simulink model "PrevVersion"  (R2020a)
settings: Solver=VariableStepAuto  StartTime=0.0  StopTime=10.0  RelTol=1e-3
libraries: simulink x3
settings Model: Creator=99003752  LastModifiedBy=99003752

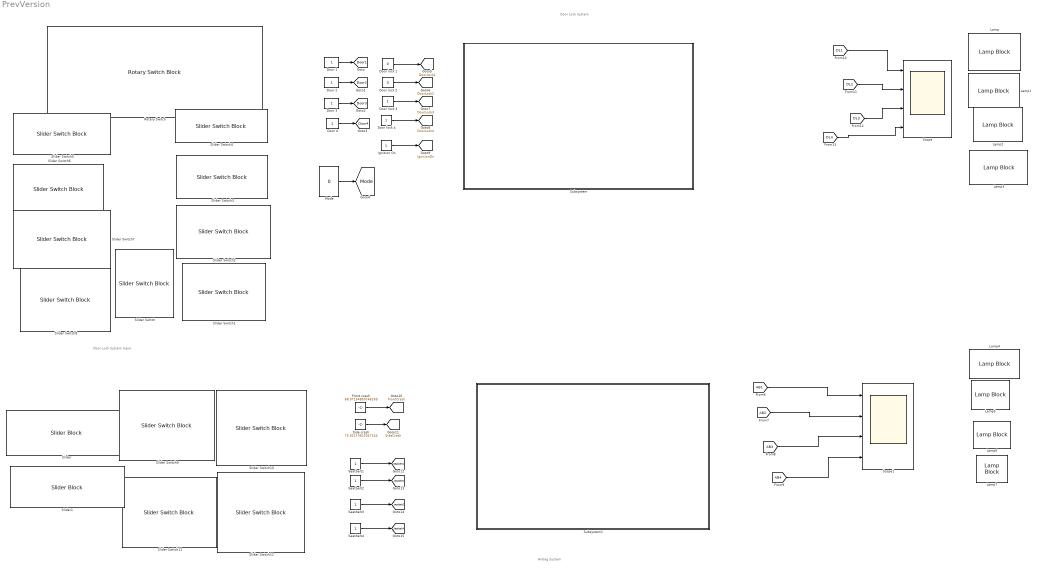
== system PrevVersion ==
  note: Door Lock System
  note: Airbag System
  note: Door Lock System Input
  Door {1..4} (4 alike) : Constant
  Door lock 1 : Constant  Value=0
  Door lock 2 : Constant  Value=0
  Door lock 3 : Constant
  Door lock 4 : Constant
  Front crash : Constant  Value=68.97154850746269
  Ignition On : Constant
  Lamp{,1..7} (8 alike) : LampBlock
  Mode : Constant  Value=0
  Rotary Switch : RotarySwitchBlock
      settings: Values={{'Off', 'Automatic Lock', 'Lock Out Protection', 'Driver Control'}, [0 1 2 3]}
  Scope : Scope  NumInputPorts=4
  Scope1 : Scope  NumInputPorts=4
  Seatbelt{1..4} (4 alike) : Constant
  Side crash : Constant  Value=75.92273622047244
  Slider : SliderBlock
  Slider Switch{,1..12} (13 alike) : SliderSwitchBlock
      settings: Values={{'Off', 'On'}, [0 1]}
  Slider1 : SliderBlock
  Subsystem : Subsystem
  Subsystem1 : Subsystem
  tag scope: Door1=global, Door2=global, Door3=global, Door4=global, DoorLock1=global, DoorLock2=global, DoorLock3=global, DoorLock4=global, FrontCrash=global, IgnitionOn=global, Mode=global, Seatbelt1=global, Seatbelt4=global, SideCrash=global, seatbelt2=global, seatbelt3=global
  wires:
  [DL4] -> Scope/4
  [DL1] -> Scope/1
  Door lock 1/1 -> [DoorLock1]
  Seatbelt1/1 -> [Seatbelt1]
  Ignition On/1 -> [IgnitionOn]
  Door lock 2/1 -> [DoorLock2]
  Door 2/1 -> [Door2]
  Door 3/1 -> [Door3]
  Seatbelt4/1 -> [Seatbelt4]
  Door lock 4/1 -> [DoorLock4]
  [DL2] -> Scope/2
  Mode/1 -> [Mode]
  Seatbelt2/1 -> [seatbelt2]
  Door 4/1 -> [Door4]
  Door lock 3/1 -> [DoorLock3]
  Seatbelt3/1 -> [seatbelt3]
  Side crash/1 -> [SideCrash]
  Front crash/1 -> [FrontCrash]
  [AB1] -> Scope1/1
  [AB2] -> Scope1/2
  Door 1/1 -> [Door1]
  [AB3] -> Scope1/3
  [DL3] -> Scope/3
  [AB4] -> Scope1/4

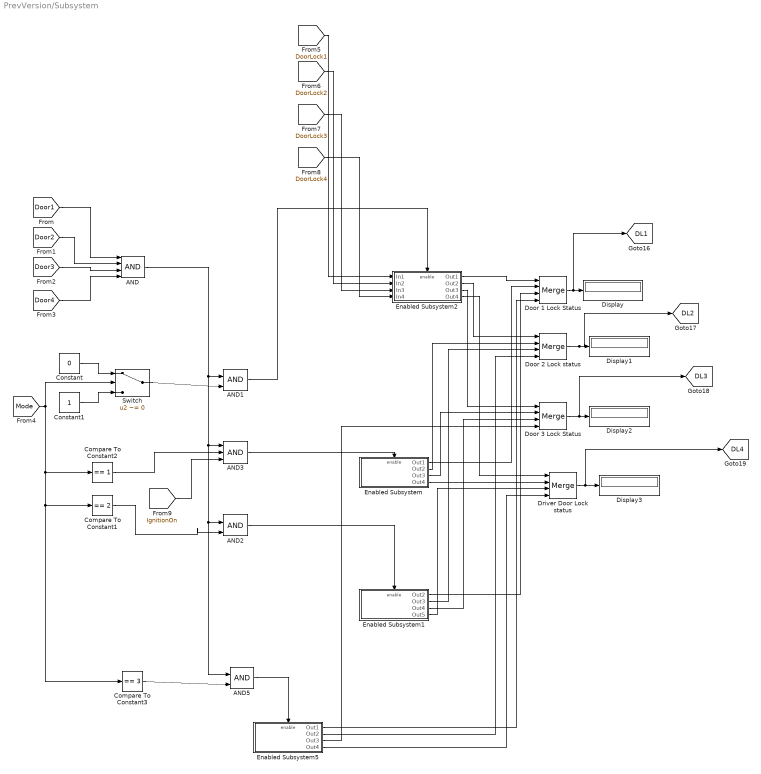
== system PrevVersion/Subsystem ==
  AND : Logic  Inputs=4  IconShape=distinctive  AllPortsSameDT=off  OutDataTypeStr=boolean
  AND1 : Logic  IconShape=distinctive  AllPortsSameDT=off  OutDataTypeStr=boolean
  AND2 : Logic  IconShape=distinctive  AllPortsSameDT=off  OutDataTypeStr=boolean
  AND3 : Logic  Inputs=3  IconShape=distinctive  AllPortsSameDT=off  OutDataTypeStr=boolean
  AND5 : Logic  IconShape=distinctive  AllPortsSameDT=off  OutDataTypeStr=boolean
  Compare To Constant1 : simulink/Logic and Bit Operations/Compare To Constant  relop===  const=2  OutDataTypeStr=boolean
  Compare To Constant2 : simulink/Logic and Bit Operations/Compare To Constant  relop===  const=1  OutDataTypeStr=boolean
  Compare To Constant3 : simulink/Logic and Bit Operations/Compare To Constant  relop===  const=3  OutDataTypeStr=boolean
  Constant : Constant  Value=0
  Constant1 : Constant
  Display{,1..3} (4 alike) : Display
  Door 1 Lock Status : Merge  Inputs=4
  Door 2 Lock status : Merge  Inputs=4
  Door 3 Lock Status : Merge  Inputs=4
  "Driver Door Lock status " : Merge  Inputs=4
  Enabled Subsystem : Subsystem  TreatAsAtomicUnit=on
  Enabled Subsystem1 : Subsystem  TreatAsAtomicUnit=on
  Enabled Subsystem2 : Subsystem  TreatAsAtomicUnit=on
  Enabled Subsystem5 : Subsystem  TreatAsAtomicUnit=on
  Switch : Switch  Criteria=u2 ~= 0
  tag scope: DL1=global, DL2=global, DL3=global, DL4=global
  wires:
  Door 1 Lock Status/1 -> [DL1], Display/1
  AND/1 -> AND5/1, AND2/1, AND3/1, AND1/1
  "Driver Door Lock status "/1 -> [DL4], Display3/1
  Door 2 Lock status/1 -> [DL2], Display1/1
  [Door4] -> AND/4
  [Mode] -> Switch/2, Compare To Constant2/1, Compare To Constant1/1, Compare To Constant3/1
  Door 3 Lock Status/1 -> [DL3], Display2/1
  Enabled Subsystem5/1(Out1) -> Door 1 Lock Status/4
  Enabled Subsystem5/2(Out2) -> Door 2 Lock status/4
  AND5/1 -> Enabled Subsystem5/Enable
  [DoorLock3] -> Enabled Subsystem2/3(In3)
  [IgnitionOn] -> AND3/3
  Enabled Subsystem1/4(Out5) -> "Driver Door Lock status "/3
  [Door1] -> AND/1
  [DoorLock4] -> Enabled Subsystem2/4(In4)
  [Door3] -> AND/3
  Enabled Subsystem2/4(Out4) -> "Driver Door Lock status "/1
  [DoorLock1] -> Enabled Subsystem2/1(In1)
  AND2/1 -> Enabled Subsystem1/Enable
  Enabled Subsystem5/3(Out3) -> Door 3 Lock Status/4
  Enabled Subsystem2/3(Out3) -> Door 3 Lock Status/1
  Enabled Subsystem5/4(Out4) -> "Driver Door Lock status "/4
  Enabled Subsystem/1(Out1) -> Door 1 Lock Status/2
  Compare To Constant3/1 -> AND5/2
  Enabled Subsystem1/2(Out3) -> Door 2 Lock status/3
  Enabled Subsystem1/1(Out2) -> Door 1 Lock Status/3
  Constant/1 -> Switch/1
  Enabled Subsystem/2(Out2) -> Door 2 Lock status/2
  Constant1/1 -> Switch/3
  AND3/1 -> Enabled Subsystem/Enable
  [Door2] -> AND/2
  Enabled Subsystem2/2(Out2) -> Door 2 Lock status/1
  Switch/1 -> AND1/2
  Enabled Subsystem/4(Out4) -> "Driver Door Lock status "/2
  Enabled Subsystem2/1(Out1) -> Door 1 Lock Status/1
  Enabled Subsystem/3(Out3) -> Door 3 Lock Status/2
  Enabled Subsystem1/3(Out4) -> Door 3 Lock Status/3
  [DoorLock2] -> Enabled Subsystem2/2(In2)
  AND1/1 -> Enabled Subsystem2/Enable
  Compare To Constant1/1 -> AND2/2
  Compare To Constant2/1 -> AND3/2

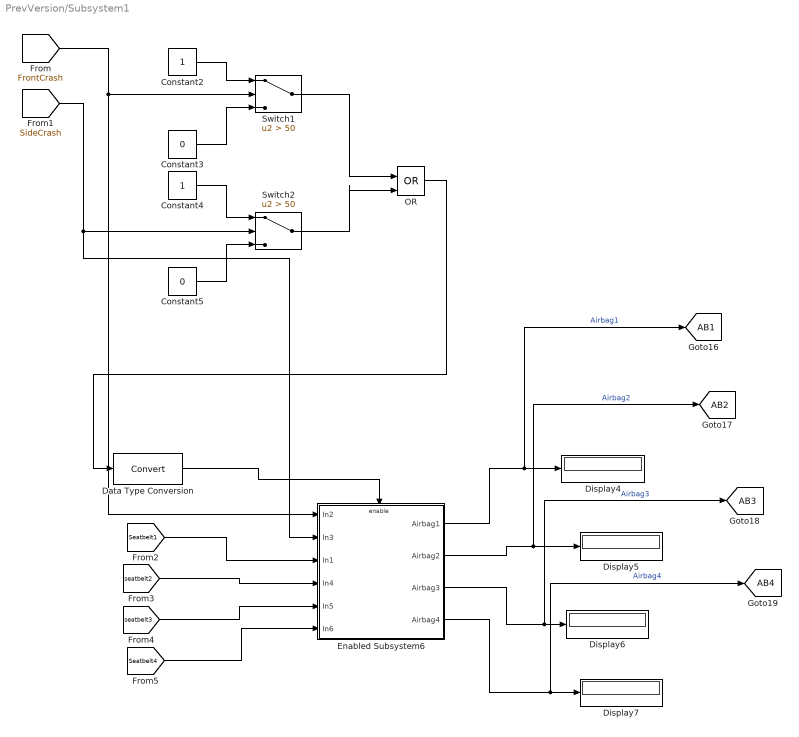
== system PrevVersion/Subsystem1 ==
  Constant2 : Constant
  Constant3 : Constant  Value=0
  Constant4 : Constant
  Constant5 : Constant  Value=0
  Data Type Conversion : DataTypeConversion
  Display{4..7} (4 alike) : Display
  Enabled Subsystem6 : Subsystem  TreatAsAtomicUnit=on
  OR : Logic  Operator=OR  IconShape=distinctive  AllPortsSameDT=off  OutDataTypeStr=boolean
  Switch1 : Switch  Criteria=u2 > Threshold  Threshold=50
  Switch2 : Switch  Criteria=u2 > Threshold  Threshold=50
  tag scope: AB1=global, AB2=global, AB3=global, AB4=global
  wires:
  Enabled Subsystem6/1(Airbag1) -> [AB1], Display4/1  "Airbag1"
  [Seatbelt4] -> Enabled Subsystem6/6(In6)
  [seatbelt3] -> Enabled Subsystem6/5(In5)
  Enabled Subsystem6/3(Airbag3) -> [AB3], Display6/1  "Airbag3"
  Enabled Subsystem6/4(Airbag4) -> [AB4], Display7/1  "Airbag4"
  Constant4/1 -> Switch2/1
  [FrontCrash] -> Enabled Subsystem6/1(In2), Switch1/2
  [Seatbelt1] -> Enabled Subsystem6/3(In1)
  Enabled Subsystem6/2(Airbag2) -> [AB2], Display5/1  "Airbag2"
  Switch2/1 -> OR/2
  Constant2/1 -> Switch1/1
  Constant3/1 -> Switch1/3
  [SideCrash] -> Enabled Subsystem6/2(In3), Switch2/2
  [seatbelt2] -> Enabled Subsystem6/4(In4)
  Data Type Conversion/1 -> Enabled Subsystem6/Enable
  Switch1/1 -> OR/1
  Constant5/1 -> Switch2/3
  OR/1 -> Data Type Conversion/1

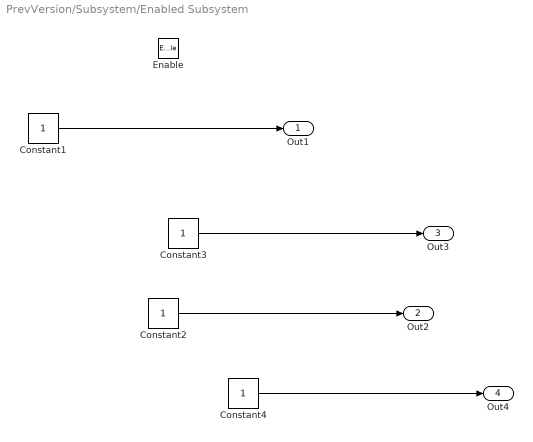
== system PrevVersion/Subsystem/Enabled Subsystem ==
  Enable : EnablePort
  Constant{1..4} (4 alike) : Constant
  Out1 : Outport
  Out2 : Outport  Port=2
  Out3 : Outport  Port=3
  Out4 : Outport  Port=4
  wires:
  Constant1/1 -> Out1/1
  Constant2/1 -> Out2/1
  Constant3/1 -> Out3/1
  Constant4/1 -> Out4/1

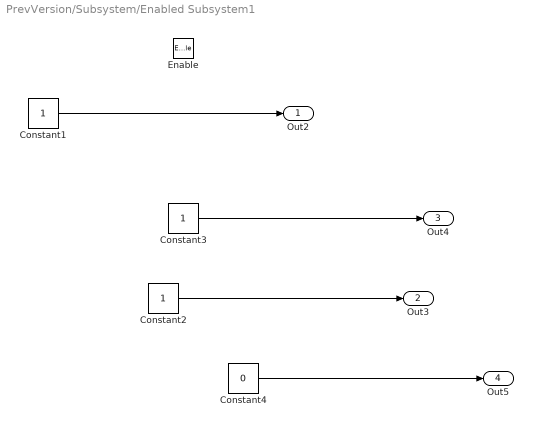
== system PrevVersion/Subsystem/Enabled Subsystem1 ==
  Enable : EnablePort
  Constant1 : Constant
  Constant2 : Constant
  Constant3 : Constant
  Constant4 : Constant  Value=0
  Out2 : Outport
  Out3 : Outport  Port=2
  Out4 : Outport  Port=3
  Out5 : Outport  Port=4
  wires:
  Constant2/1 -> Out3/1
  Constant3/1 -> Out4/1
  Constant1/1 -> Out2/1
  Constant4/1 -> Out5/1

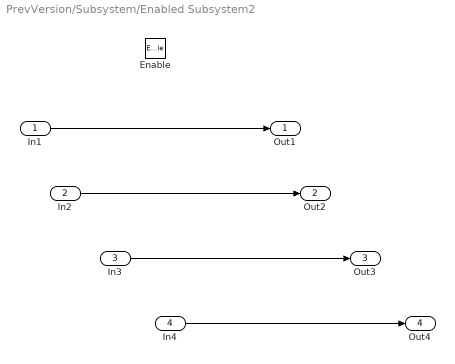
== system PrevVersion/Subsystem/Enabled Subsystem2 ==
  In1 : Inport
  In2 : Inport  Port=2
  In3 : Inport  Port=3
  In4 : Inport  Port=4
  Enable : EnablePort
  Out1 : Outport
  Out2 : Outport  Port=2
  Out3 : Outport  Port=3
  Out4 : Outport  Port=4
  wires:
  In1/1 -> Out1/1
  In2/1 -> Out2/1
  In3/1 -> Out3/1
  In4/1 -> Out4/1

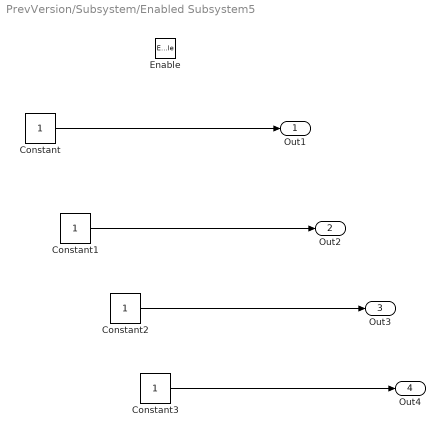
== system PrevVersion/Subsystem/Enabled Subsystem5 ==
  Enable : EnablePort
  Constant{,1..3} (4 alike) : Constant
  Out1 : Outport
  Out2 : Outport  Port=2
  Out3 : Outport  Port=3
  Out4 : Outport  Port=4
  wires:
  Constant/1 -> Out1/1
  Constant1/1 -> Out2/1
  Constant2/1 -> Out3/1
  Constant3/1 -> Out4/1

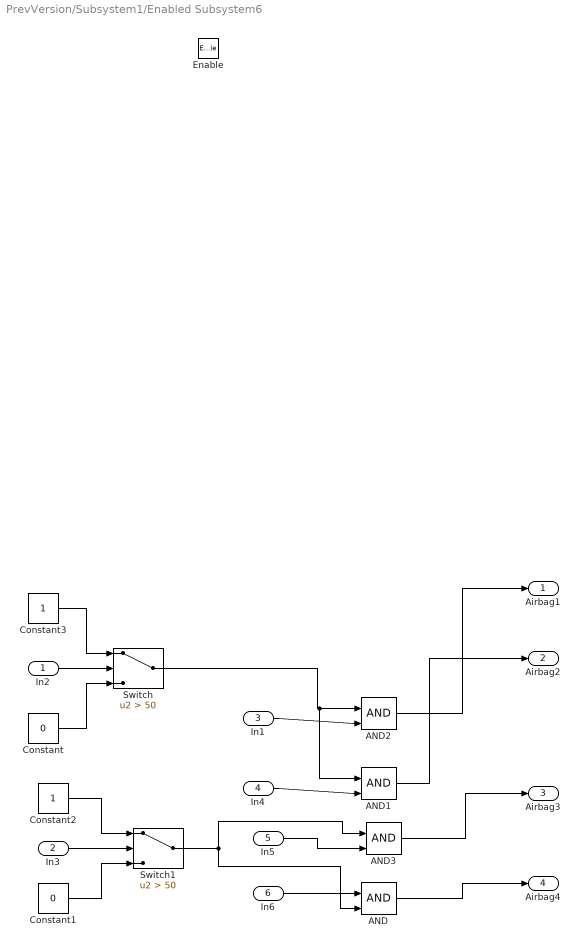
== system PrevVersion/Subsystem1/Enabled Subsystem6 ==
  In2 : Inport
  In3 : Inport  Port=2
  In1 : Inport  Port=3
  In4 : Inport  Port=4
  In5 : Inport  Port=5
  In6 : Inport  Port=6
  Enable : EnablePort
  AND{,1..3} (4 alike) : Logic  IconShape=distinctive  AllPortsSameDT=off  OutDataTypeStr=boolean
  Constant : Constant  Value=0
  Constant1 : Constant  Value=0
  Constant2 : Constant
  Constant3 : Constant
  Switch : Switch  Criteria=u2 > Threshold  Threshold=50
  Switch1 : Switch  Criteria=u2 > Threshold  Threshold=50
  Airbag1 : Outport
  Airbag2 : Outport  Port=2
  Airbag3 : Outport  Port=3
  Airbag4 : Outport  Port=4
  wires:
  Constant2/1 -> Switch1/1
  In2/1 -> Switch/2
  Constant/1 -> Switch/3
  In3/1 -> Switch1/2
  Constant1/1 -> Switch1/3
  Constant3/1 -> Switch/1
  In1/1 -> AND2/2
  In4/1 -> AND1/2
  In6/1 -> AND/1
  In5/1 -> AND3/2
  Switch/1 -> AND1/1, AND2/1
  AND2/1 -> Airbag1/1
  AND1/1 -> Airbag2/1
  AND3/1 -> Airbag3/1
  AND/1 -> Airbag4/1
  Switch1/1 -> AND/2, AND3/1
